simulink model "compensacion_analogica"  (R2014b)
settings: Solver=ode45  StartTime=0.0  StopTime=4  RelTol=1e-3
settings Model: Creator=Javi  LastModifiedBy=Javi

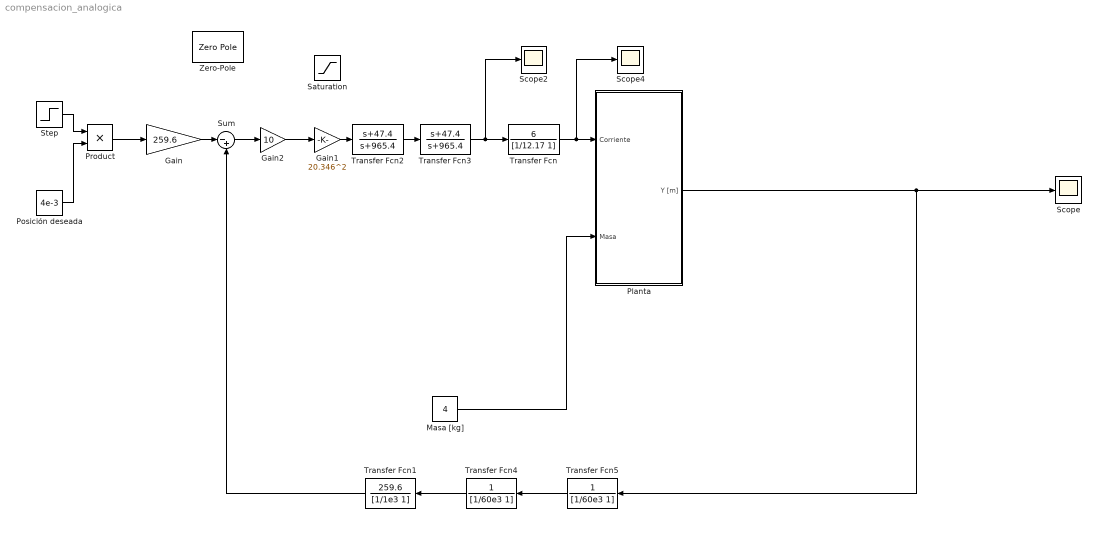
== system compensacion_analogica ==
  Gain : Gain  Gain=259.6
  Gain1 : Gain  Gain=20.346^2
  Gain2 : Gain  Gain=10
  "Masa [kg] " : Constant  Value=4
  "Planta " : Subsystem
  Posición deseada : Constant  Value=4e-3
  Product : Product
  Saturation : Saturate  UpperLimit=5  LowerLimit=-inf
  Scope : Scope
      settings: TimeRange=4  YMin=0  YMax=0.014
  Scope2 : Scope
      settings: TimeRange=0.005185185185185187  YMin=-3500000  YMax=500000  SaveName=ScopeData2
  Scope4 : Scope
      settings: TimeRange=0.005185185185185187  YMin=-3500000  YMax=500000  SaveName=ScopeData4
  Step : Step  Time=0.01  SampleTime=0
  Sum : Sum  Inputs=|-+
  Transfer Fcn : TransferFcn  Numerator=[6]  Denominator=[1/12.17 1]
  Transfer Fcn1 : TransferFcn  Numerator=259.6  Denominator=[1/1e3 1]
  Transfer Fcn2 : TransferFcn  Numerator=[1 47.4]  Denominator=[1 965.4]
  Transfer Fcn3 : TransferFcn  Numerator=[1 47.4]  Denominator=[1 965.4]
  Transfer Fcn4 : TransferFcn  Numerator=1  Denominator=[1/60e3 1]
  Transfer Fcn5 : TransferFcn  Numerator=1  Denominator=[1/60e3 1]
  Zero-Pole : ZeroPole  Zeros=[-221.7 -221.7]  Poles=[-4511 -4511]  Gain=8.28e5
  wires:
  "Masa [kg] "/1 -> "Planta "/2("Masa ")
  "Planta "/1(Y [m]) -> Scope/1, Transfer Fcn5/1
  Gain/1 -> Sum/1
  Transfer Fcn1/1 -> Sum/2
  Transfer Fcn/1 -> "Planta "/1(Corriente), Scope4/1
  Transfer Fcn3/1 -> Scope2/1, Transfer Fcn/1
  Step/1 -> Product/1
  Posición deseada/1 -> Product/2
  Product/1 -> Gain/1
  Transfer Fcn2/1 -> Transfer Fcn3/1
  Gain1/1 -> Transfer Fcn2/1
  Sum/1 -> Gain2/1
  Gain2/1 -> Gain1/1
  Transfer Fcn4/1 -> Transfer Fcn1/1
  Transfer Fcn5/1 -> Transfer Fcn4/1

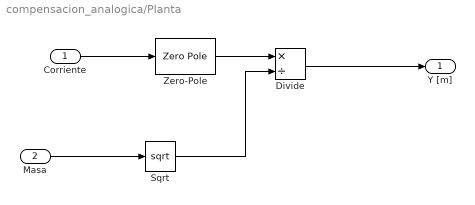
== system compensacion_analogica/Planta  ==
  Corriente : Inport
  "Masa " : Inport  Port=2
  Divide : Product  Inputs=*/
  Sqrt : Sqrt  SaturateOnIntegerOverflow=on
  Zero-Pole : ZeroPole  Zeros=[]  Poles=[70 -70]  Gain=-6.58
  Y [m] : Outport
  wires:
  Divide/1 -> Y [m]/1
  Corriente/1 -> Zero-Pole/1
  Zero-Pole/1 -> Divide/1
  "Masa "/1 -> Sqrt/1
  Sqrt/1 -> Divide/2
